simulink subsystem "s0328_static_motor_simulator"  (R2019b)
settings: Solver=VariableStepAuto  StartTime=0.0  StopTime=10.0  RelTol=1e-3
model mask{omega_0=0, i_0=0}
  mask prompts: omega_0 "Initial Speed"; i_0 "Initial Current"
undefined symbols (not defined in the file): PARAMS
settings Model: Creator=paolo  LastModifiedBy=alessandro
settings DebuggingCC: SFMachineParentedDataDiag=error

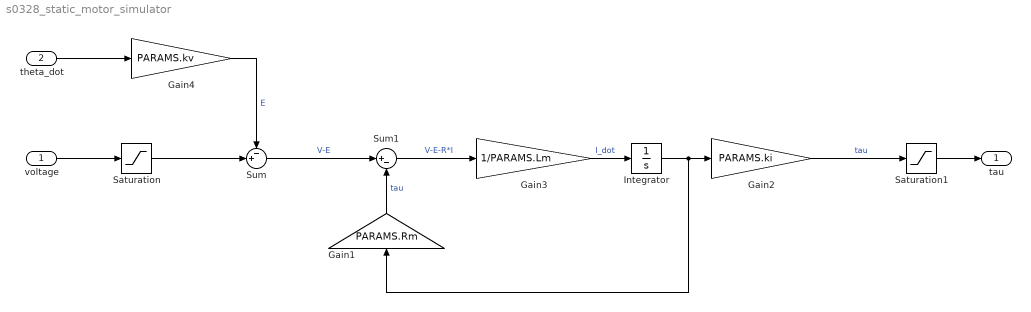
== system s0328_static_motor_simulator ==
  voltage : Inport
  theta_dot : Inport  Port=2
  Gain1 : Gain  Gain=PARAMS.Rm
  Gain2 : Gain  Gain=PARAMS.ki
  Gain3 : Gain  Gain=1/PARAMS.Lm
  Gain4 : Gain  Gain=PARAMS.kv
  Integrator : Integrator
  Saturation : Saturate  UpperLimit=PARAMS.V_sat  LowerLimit=-PARAMS.V_sat
  Saturation1 : Saturate  UpperLimit=PARAMS.tau_nom  LowerLimit=-PARAMS.tau_nom
  Sum : Sum  Inputs=-+|
  Sum1 : Sum  Inputs=|+-
  tau : Outport
  wires:
  voltage/1 -> Saturation/1
  Gain4/1 -> Sum/1  "E"
  theta_dot/1 -> Gain4/1
  Saturation/1 -> Sum/2
  Gain2/1 -> Saturation1/1  "tau"
  Saturation1/1 -> tau/1
  Sum/1 -> Sum1/1  "V-E"
  Integrator/1 -> Gain2/1, Gain1/1
  Gain1/1 -> Sum1/2  "tau"
  Sum1/1 -> Gain3/1  "V-E-R*I"
  Gain3/1 -> Integrator/1  "I_dot"
